simulink model "Model_plane6_new_land_animation"  (R2024a)
settings: Solver=FixedStepAuto  StartTime=0  StopTime=600  FixedStep=0.01  RelTol=1e-3
model workspace (MAT data in the model file):
  Alfa = [-2 4 10 16]
  Alfa_RUD = 0.55
  Alfa_table = [-4 0 5 10 20]
  Alfa_y = [-4 6 8 9 10 12 14]
  Cxa_table = [0.03434 0.02598 0.04151 0.122 0.502 0.0358 0.0252 0.0505 0.1649 0.538 0.04274 0.0262 ... (15 elements, 5x3)]
  Cy_DB = [0.01242 0.01286 0.01457]
  Cy_fi = [0.00623 0.00643 0.00626]
  Cya = [-0.276 0.859 1.085 1.2 1.296 1.45 1.461 -0.33 0.991 1.211 1.275 1.29 ... (21 elements, 7x3)]
  Del_B = -5
  H = [339 3256 4060 8000 12000]
  H_table = [0 2000 4000 6000 8000 10000]
  I = [1000 1000 4500000]
  K_dH = -0.3
  K_p = 0.3
  K_roll = 1
  K_w = 1.5
  K_wx = 1
  K_wy = 1
  Ki_H = 1e-05
  Ki_P = 1
  Ki_V = 0.009
  Ki_n = 1
  Kp_H = 0.03
  Kp_P = 1
  Kp_V = 0.9
  Kp_n = 1
  M_C = [0.4 0.6 0.82]
  M_mz = [0.2 0.4 0.6 0.8]
  M_mz2 = [0.4 0.7 0.85]
  M_table = [0.4 0.7 0.82]
  M_y = [0.4 0.7 0.82]
  P = [70000 56000 44800 35840 28672]
  Psi0 = 0
  Skr = 131
  Teta0 = 0
  V0 = 135
  a_table = [340.3 339.5 338.8 338 337.2 336.4]
  ba = 3.466
  fi = 0
  fi_P = 2
  g = 9.81
  lz = 4500000
  mla = 60000
  mz_DB = [-0.035 -0.0358 -0.037 -0.0377]
  mz_alfa = [-0.0282 -0.0282 -0.0289 -0.0404]
  mz_alfa2 = [-8.163  -8.762  -9.714; -8.163  -8.762  -9.583; -7.975  -7.991  -7.868; -6.514  -6.413  -6.732]
  mz_fi = [-0.0695 -0.0714 -0.0739 -0.0832]
  mz_omz = [-23.768  -25.3  -28.284; -23.768  -25.3  -27.903; -23.222  -22.6  -23.32; -18.967  -18.52  -19.601]
  n_dvig = 2
  out : Simulink.SimulationOutput (value not decoded)
  pitch = 1
  pitch0 = 0
  q_table = [1.225 1.0065 0.8194 0.6601 0.5258 0.4135]
  roll0 = 0
  wx0 = 0
  wy0 = 0
  wz0 = 0
  x0 = 0
  xy = [240000 6200]
  y0 = 1000
  yaw0 = 0
  z0 = 0
libraries: simulink x13, sim3dlib x2, aerolibsim3d x1
(part 2 of 2)

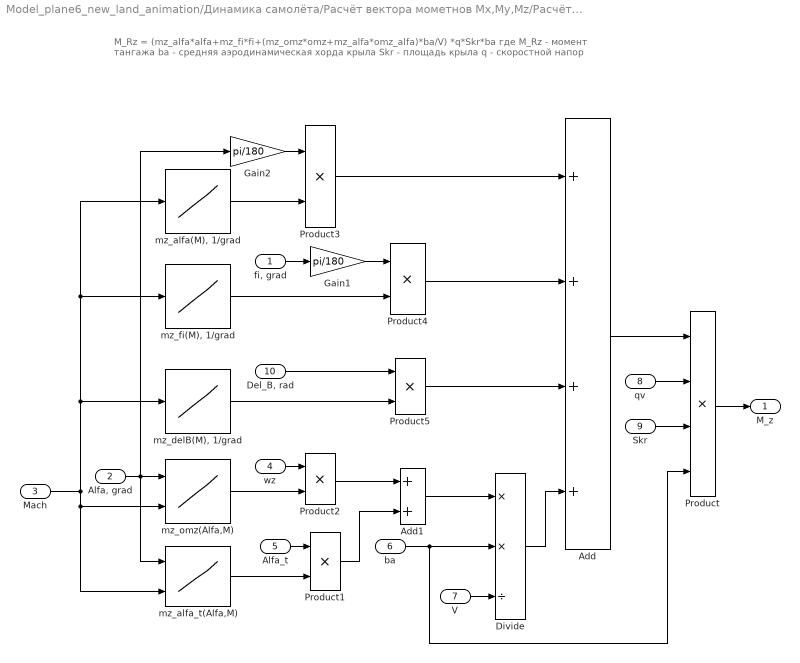
== system Model_plane6_new_land_animation/Динамика самолёта/Расчёт вектора мометнов Mx,My,Mz/Расчёт M_z (момент тангажа) ==
  note: M_Rz = (mz_alfa*alfa+mz_fi*fi+(mz_omz*omz+mz_alfa*omz_alfa)*ba/V) *q*Skr*ba
      | где M_Rz - момент тангажа
      | ba - средняя аэродинамическая хорда крыла
      | Skr - площадь крыла
      | q - скоростной напор
  "fi, grad" : Inport
  "Alfa, grad" : Inport  Port=2
  Mach : Inport  Port=3
  wz : Inport  Port=4
  Alfa_t : Inport  Port=5
  ba : Inport  Port=6
  V : Inport  Port=7
  qv : Inport  Port=8
  Skr : Inport  Port=9
  "Del_B, rad" : Inport  Port=10
  Add : Sum  Inputs=++++
  Add1 : Sum
  Divide : Product  Inputs=**/
  Gain1 : Gain  Gain=pi/180
  Gain2 : Gain  Gain=pi/180
  Product : Product  Inputs=4
  Product{1..5} (5 alike) : Product
  "mz_alfa(M), 1/grad" : Lookup_n-D  NumberOfTableDimensions=1  BreakpointsForDimension1=M_mz  Table=mz_alfa  InternalRulePriority=Speed  RndMeth=Simplest
  mz_alfa_t(Alfa,M) : Lookup_n-D  BreakpointsForDimension1=Alfa  BreakpointsForDimension2=M_mz2  Table=mz_alfa2  InternalRulePriority=Speed  RndMeth=Simplest
      settings: InputPortMap=u0,u1
  "mz_delB(M), 1/grad" : Lookup_n-D  NumberOfTableDimensions=1  BreakpointsForDimension1=M_mz  Table=mz_DB  InternalRulePriority=Speed  RndMeth=Simplest
  "mz_fi(M), 1/grad" : Lookup_n-D  NumberOfTableDimensions=1  BreakpointsForDimension1=M_mz  Table=mz_fi  InternalRulePriority=Speed  RndMeth=Simplest
  mz_omz(Alfa,M) : Lookup_n-D  BreakpointsForDimension1=Alfa  BreakpointsForDimension2=M_mz2  Table=mz_omz  InternalRulePriority=Speed  RndMeth=Simplest
      settings: InputPortMap=u0,u1
  M_z : Outport
  wires:
  Product/1 -> M_z/1
  ba/1 -> Product/4, Divide/2
  Skr/1 -> Product/3
  qv/1 -> Product/2
  Add/1 -> Product/1
  V/1 -> Divide/3
  Divide/1 -> Add/4
  Add1/1 -> Divide/1
  Product2/1 -> Add1/1
  Product1/1 -> Add1/2
  Alfa_t/1 -> Product1/1
  wz/1 -> Product2/1
  mz_omz(Alfa,M)/1 -> Product2/2
  mz_alfa_t(Alfa,M)/1 -> Product1/2
  Mach/1 -> mz_omz(Alfa,M)/2, mz_alfa_t(Alfa,M)/2, "mz_alfa(M), 1/grad"/1, "mz_fi(M), 1/grad"/1, "mz_delB(M), 1/grad"/1
  "mz_alfa(M), 1/grad"/1 -> Product3/2
  "mz_fi(M), 1/grad"/1 -> Product4/2
  Product3/1 -> Add/1
  Product4/1 -> Add/2
  Product5/1 -> Add/3
  "Del_B, rad"/1 -> Product5/1
  "fi, grad"/1 -> Gain1/1
  Gain1/1 -> Product4/1
  "Alfa, grad"/1 -> Gain2/1, mz_omz(Alfa,M)/1, mz_alfa_t(Alfa,M)/1
  Gain2/1 -> Product3/1
  "mz_delB(M), 1/grad"/1 -> Product5/2

== matlab function Model_plane6_new_land_animation/Динамика самолёта/Расчёт вектора мометнов Mx,My,Mz/Вектор моментов ==
  data: M_x input; M output; M_y input; M_z input
function M = fcn(M_x, M_y, M_z)

M=[M_x; M_y; M_z];

== matlab function Model_plane6_new_land_animation/Динамика самолёта/Вектор состояния/Расчёт скорости ==
  data: Fkx input; dV output; mla input
function dV = fcn(Fkx, mla)

dV=Fkx/mla;

== matlab function Model_plane6_new_land_animation/Динамика самолёта/Вектор состояния/Рассчёт скоростей в земной СК ==
  data: V input; dx output; Teta input; Psi input; dy output; dz output
function [dx, dy, dz] = fcn(V, Teta, Psi)

dx=V*cos(Psi)*cos(Teta);
dy=V*sin(Teta);
dz=-V*sin(Psi)*cos(Teta);

== matlab function Model_plane6_new_land_animation/Динамика самолёта/Вектор состояния/Рассчёт углового измнения момента wx ==
  data: Mx input; dwx output; I input; wy input; wz input
function dwx = fcn(Mx,I,wy,wz)

dwx=(Mx-(I(3)-I(2))*wy*wz)/I(1);

== matlab function Model_plane6_new_land_animation/Динамика самолёта/Вектор состояния/Рассчёт изменения угла рыскания ==
  data: dyaw output; wy input; wz input; pitch input; roll input
function dyaw = fcn(wy,wz,pitch,roll)

dyaw=(wy*cos(roll)-wz*sin(roll))/cos(pitch);

== matlab function Model_plane6_new_land_animation/Динамика самолёта/Вектор состояния/Вектор состояния ==
  data: dV input; S output; dTeta input; dPsi input; dxg input; dyg input; dzg input; dwx input; dwy input; dwz input; dyaw input; dpitch input; droll input
function S = fcn(dV,dTeta,dPsi,dxg,dyg,dzg,dwx,dwy,dwz,dyaw,dpitch,droll)

S=[dV;dTeta;dPsi;dxg;dyg;dzg;dwx;dwy;dwz;dyaw;dpitch;droll];

== matlab function Model_plane6_new_land_animation/Динамика самолёта/Вектор состояния/Координаты положения в пространстве ==
  data: xg input; xyz output; yg input; zg input
function xyz = fcn(xg,yg,zg)

xyz=[xg;yg;zg];

== matlab function Model_plane6_new_land_animation/Динамика самолёта/Вектор состояния/Вектор угловых скоростей ==
  data: wx input; w output; wy input; wz input
function w = fcn(wx,wy,wz)

w=[wx;wy;wz];

== matlab function Model_plane6_new_land_animation/Динамика самолёта/Вектор состояния/Углы положения в пространстве ==
  data: roll input; pitch input; yaw input; rpy output
function rpy = fcn(roll,pitch,yaw)

rpy=[roll;pitch;yaw];

== matlab function Model_plane6_new_land_animation/Динамика самолёта/Вектор состояния/Вектор V, Teta, Psi ==
  data: V input; VTP output; Teta input; Psi input
function VTP = fcn(V,Teta,Psi)

VTP=[V;Teta;Psi];

== matlab function Model_plane6_new_land_animation/Динамика самолёта/Рассчёт вектора аэродинамических сил/Вектор аэродинамических сил ==
  data: Xa input; A output; Ya input; Za input
function A = fcn(Xa, Ya, Za)

A=[Xa;Ya;Za];

== matlab function Model_plane6_new_land_animation/Динамика самолёта/Вектор состояния/MATLAB Function1 ==
  data: Teta input; Alfa output; pitch input; yaw input; Psi input; Beta output; roll input
function [Alfa, Beta] = fcn(Teta, pitch, yaw, Psi,roll)
%Alfa=pitch-Teta;
%Beta=yaw-Psi;

Alfa=-atan((sin(roll)*cos(Teta)*sin(yaw-Psi)-cos(roll)*sin(pitch)*cos(Teta)*cos(yaw-Psi)+cos(roll)*cos(pitch)*sin(Teta))/(cos(pitch)*cos(Teta)*cos(yaw-Psi)+sin(pitch)*sin(Teta)));
Beta=asin(cos(roll)*cos(Teta)*sin(yaw-Psi)+sin(roll)*sin(pitch)*cos(Teta)*cos(yaw-Psi)-sin(roll)*cos(pitch)*sin(Teta));

== matlab function Model_plane6_new_land_animation/Динамика самолёта/Вектор состояния/Рассчёт угла наклона траектории ==
  data: Fky input; dTeta output; V input; mla input
function dTeta = fcn(Fky,V,mla)

dTeta=Fky/(mla*V);

== matlab function Model_plane6_new_land_animation/Динамика самолёта/Вектор состояния/Расчёт угла пути ==
  data: Fkz input; dPsi output; mla input; V input; Teta input
function dPsi = fcn(Fkz,mla,V,Teta)
dPsi=-Fkz/(mla*V*cos(Teta));

== matlab function Model_plane6_new_land_animation/Динамика самолёта/Вектор состояния/Рассчёт углового измнения момента wy ==
  data: My input; I input; wx input; wz input; dwy output
function dwy = fcn(My,I,wx,wz)

dwy=(My-(I(1)-I(2))*wx*wz)/I(2);

== matlab function Model_plane6_new_land_animation/Динамика самолёта/Вектор состояния/Рассчёт углового измнения момента wz ==
  data: Mz input; I input; wx input; wy input; dwz output
function dwz = fcn(Mz,I,wx,wy)

dwz=(Mz-(I(2)-I(1))*wx*wy)/I(3);

== matlab function Model_plane6_new_land_animation/Динамика самолёта/Вектор состояния/Рассчёт изменения угла тангажа ==
  data: wy input; wz input; roll input; dpitch output
function dpitch = fcn(wy,wz,roll)

dpitch=wy*sin(roll)+wz*cos(roll);

== matlab function Model_plane6_new_land_animation/Динамика самолёта/Вектор состояния/Рассчёт изменения угла крена ==
  data: wx input; wy input; wz input; pitch input; roll input; droll output
function droll = fcn(wx,wy,wz,pitch,roll)

droll=wx-(wy*cos(roll)-wz*sin(roll))*tan(pitch);

== matlab function Model_plane6_new_land_animation/Динамика самолёта/Расчёт вектора мометнов Mx,My,Mz/Расчёт M_y (момент рыскания)/MATLAB Function ==
  data: u input; M_y output
function M_y = fcn(u)
c=0;

M_y = c*u;

== matlab function Model_plane6_new_land_animation/Динамика самолёта/Вектор состояния/MATLAB Function2 ==
  data: pitch input; roll_a output; Alfa input; roll input; Teta input; Beta input
function roll_a = fcn(pitch,Alfa,roll,Teta,Beta)

roll_a=asin((sin(pitch)*cos(Alfa)*sin(Beta)-cos(roll)*cos(pitch)*sin(Alfa)*sin(Beta)+sin(roll)*cos(pitch)*cos(Beta))/cos(Teta));

== matlab function Model_plane6_new_land_animation/Динамика самолёта/Рассчёт вектора аэродинамических сил/Расчёт Za (бокового воздействия)/MATLAB Function ==
  data: qv input; Za output; Skr input
function Za = fcn(qv,Skr)
Cz=0;

Za=Cz*qv*Skr;

== matlab function Model_plane6_new_land_animation/Динамика самолёта/Вектор состояния/MATLAB Function3 ==
  data: V input; Vx output; Alfa input
function Vx = fcn(V,Alfa)

Vx=sqrt(V^2/(1+(tan(-Alfa))^2));

== matlab function Model_plane6_new_land_animation/If Action Subsystem1/MATLAB Function ==
  data: y_const input; H output; v_const input; V output
function [H, V] = fcn(y_const, v_const)
%#codegen

H = y_const;
V = v_const;

== matlab function Model_plane6_new_land_animation/Динамика самолёта/MATLAB Function ==
  data: wx input; roll input; wy input; Psi input; nz input; V input; U output; y input; dy input; pitch input; w_z input
function U = fcn(wx, roll,wy,Psi,nz, V,y,dy,pitch,w_z)

U=[wx,roll,wy,Psi, nz, V,y,dy,pitch,w_z];

== matlab function Model_plane6_new_land_animation/If Action Subsystem/Выдерживание/MATLAB Function ==
  data: H output; mla input; g input; Skr input; ro input; V_p output; cy_p input; alfa input
function [H,V_p] = fcn(mla,g,Skr,ro, cy_p, alfa)



if (alfa*180/pi<8)
    H=3;
else 
    H=0;
end

V_p=0.09*(sqrt((2*mla*g)/(cy_p*ro*Skr)));
%V_p=25;

== matlab function Model_plane6_new_land_animation/If Action Subsystem/Планирование/MATLAB Function ==
  data: H output; mla input; g input; Skr input; ro input; V_zp output; c_y input
function [H,V_zp] = fcn(mla,g,Skr,ro, c_y)
%c_y=1.9;
H=5;
V_zp=0.45*(sqrt((2*mla*g)/(c_y*ro*Skr)));

== matlab function Model_plane6_new_land_animation/If Action Subsystem/If Action Subsystem2/MATLAB Function ==
  data: H output; V_p output
function [H,V_p] = fcn()
H=0;
V_p=0;
%V_p=25;

== matlab function Model_plane6_new_land_animation/Динамика самолёта/Рассчёт перегрузок/MATLAB Function ==
  data: Fx input; Fy input; Fz input; n output; mla input; g input
function n = fcn(Fx,Fy, Fz, mla,g)

nx=Fx/mla*g;
ny=Fy/mla*g;
nz=Fz/mla*g;

n=[nx,ny,nz];

== matlab function Model_plane6_new_land_animation/Динамика самолёта/Вектор тяги двигателя/Вектор тяги ==
  data: Px input; P output; Py input
function P = fcn(Px,Py)

P=[Px;Py;0];

== matlab function Model_plane6_new_land_animation/Динамика самолёта/Вектор внешних сил/MATLAB Function ==
  data: mla input; l input; W output; g input; k input; Vy input
function W = fcn(mla,l,g,k, Vy)
if l==0
    b=0;
else
    b=0.7;
end

W=[-k*mla*g; (l*mla*g+b*Vy); 0];

== matlab function Model_plane6_new_land_animation/Динамика самолёта/Вектор проекций аэродинамических сил/MATLAB Function ==
  data: A input; Fk output; P input; W input; Teta input; Psi input; Alfa input; Beta input; roll_a input; yaw input; pitch input; roll input
function Fk = fcn(A,P,W,Teta,Psi,Alfa,Beta,roll_a,yaw,pitch,roll)

yaw_a=Psi;
pitch_a=Teta;


D_g_k = [cos(Psi)*cos(Teta), sin(Teta), -sin(Psi)*cos(Teta);
        -cos(Psi)*sin(Teta), cos(Teta), sin(Psi)*sin(Teta);
        sin(Psi), 0, cos(Psi)];

D_gv = [cos(yaw_a)*cos(pitch_a), sin(pitch_a), -sin(yaw_a)*cos(pitch_a);
        -cos(yaw_a)*sin(pitch_a)*cos(roll_a) + sin(yaw_a)*sin(roll_a), cos(pitch_a)*cos(roll_a), cos(yaw_a)*sin(roll_a) + sin(yaw_a)*sin(pitch_a)*cos(roll_a);
        cos(yaw_a)*sin(pitch_a)*sin(roll_a) + sin(yaw_a)*cos(roll_a), -cos(pitch_a)*sin(roll_a), cos(yaw_a)*cos(roll_a) - sin(yaw_a)*sin(pitch_a)*sin(roll_a)];
 
D_g_cv=[cos(yaw)*cos(pitch), sin(pitch), -sin(yaw)*cos(pitch);
    sin(yaw)*sin(roll)-cos(yaw)*sin(pitch)*cos(roll), cos(pitch)*cos(roll), cos(yaw)*sin(roll)+sin(yaw)*sin(pitch)*cos(roll);
    sin(yaw)*cos(roll)+cos(yaw)*sin(pitch)*sin(roll), -cos(pitch)*sin(roll), cos(yaw)*cos(roll)-sin(yaw)*sin(pitch)*sin(roll)];

D_cv_a = [cos(Alfa)*cos(Beta), -sin(Alfa)*cos(Beta), sin(Beta);
        sin(Alfa), cos(Alfa), 0;
        -cos(Alfa)*sin(Beta), sin(Alfa)*sin(Beta), cos(Beta)];

Fk = D_g_k * (D_g_cv' * (D_cv_a' * A + P) + W);

== matlab function Model_plane6_new_land_animation/Динамика самолёта/Блок расчёта параметров стандартной атмосферы/MATLAB Function ==
  data: ro input; a input; q output; V input; M output
function [q, M] = fcn(ro, a, V)

q=(ro*V^2)/2;
M=V/a;

== matlab function Model_plane6_new_land_animation/Динамика самолёта/Расчёт вектора мометнов Mx,My,Mz/Расчёт M_x (момент крена)/MATLAB Function ==
  data: u input; M_x output
function M_x = fcn(u)
c=0;

M_x = c*u;

== matlab function Model_plane6_new_land_animation/Динамика самолёта/Вектор тяги двигателя/Проекции аэродинамических сил ==
  data: Px output; fi_p input; P input; alfa_Rud input; n_dvig input; Py output
function [Px, Py] = fcn(fi_p,P,alfa_Rud,n_dvig)

Px=cos(fi_p)*(n_dvig*alfa_Rud*P);
Py=sin(fi_p)*(n_dvig*alfa_Rud*P);
